simulink model "untitled1"  (R2013a)
settings: Solver=ode45  StartTime=0.0  StopTime=10  RelTol=1e-3
values from neighbouring files (symbols this model uses):
  A = [0 1 0 0 ... (first row only)    [Untitled.m]    (also in Untitled102.m = [0,1,0,0;0,0.2,2,-0.6;0,0,0,1;0,2,5,8]; lqr.m = [0,1,0,0;0,-126.3,-12.8,5.1;0,0,0,1;0,1446.9,213.6,-57.9])
  B = [ 0 ... (first row only)    [Untitled.m]    (also in Untitled102.m = [0;2;5;2]; lqr.m = [0;10.7;0;-122.6])
  C = eye(4)    [Untitled.m]    (also in Untitled102.m = [0,0,1,0:0,0,0,1]; lqr.m = [0,0,1,0;0,0,0,1])
settings Model: Creator=user  LastModifiedBy=user

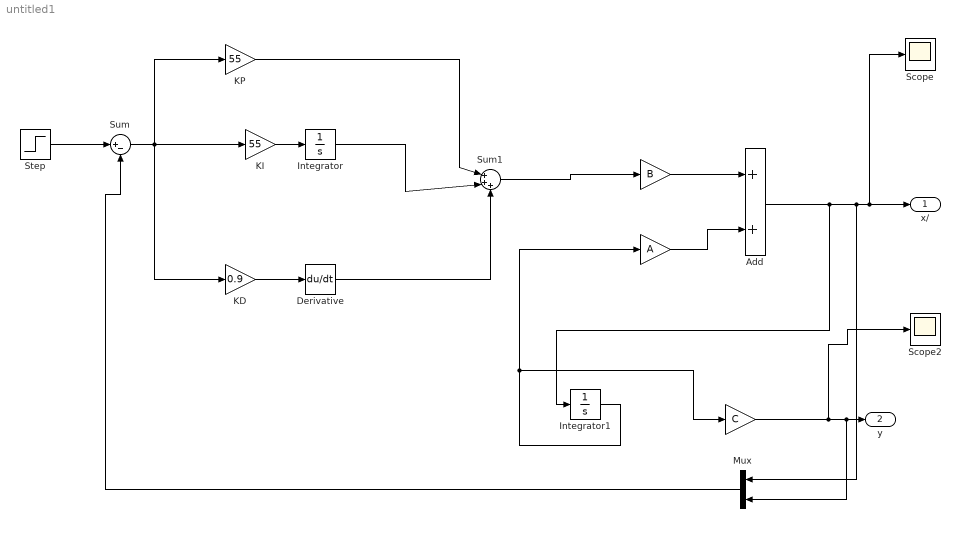
== system untitled1 ==
  " " : Gain  Gain=B
  " " : Gain  Gain=A
  " " : Gain  Gain=C
  Add : Sum
  Derivative : Derivative
  Integrator : Integrator
  Integrator1 : Integrator
  KD : Gain  Gain=0.9
  KI : Gain  Gain=55
  KP : Gain  Gain=55
  Mux : Mux  Inputs=2
  Scope : Scope
  Scope2 : Scope
      settings: SaveName=ScopeData2
  Step : Step  After=90  SampleTime=1
  Sum : Sum  Inputs=|+-
  Sum1 : Sum  Inputs=|+++
  "x/ " : Outport
  y : Outport  Port=2
  wires:
  KP/1 -> Sum1/1
  Integrator/1 -> Sum1/2
  Derivative/1 -> Sum1/3
  Sum/1 -> KD/1, KI/1, KP/1
  KI/1 -> Integrator/1
  KD/1 -> Derivative/1
  " "/1 -> Add/1
  " "/1 -> Add/2
  " "/1 -> Scope2/1, Mux/2, y/1
  Sum1/1 -> " "/1
  Add/1 -> Integrator1/1, Mux/1, Scope/1, "x/ "/1
  Integrator1/1 -> " "/1, " "/1
  Step/1 -> Sum/1
  Mux/1 -> Sum/2
